simulink model "Control_Pc_prueba"  (R2021b)
settings: Solver=FixedStepDiscrete  StartTime=0.0  StopTime=inf  FixedStep=0.01  MaxStep=0.01  RelTol=1e-3
InitFcn:
  | Ts=0.01;
libraries: instrumentseriallib x2
settings Model: Creator=eva_g  LastModifiedBy=Laura Sierra Ruiz
settings SolverCC: AlgebraicLoopSolver=TrustRegion
settings DebuggingCC: SFMachineParentedDataDiag=warning

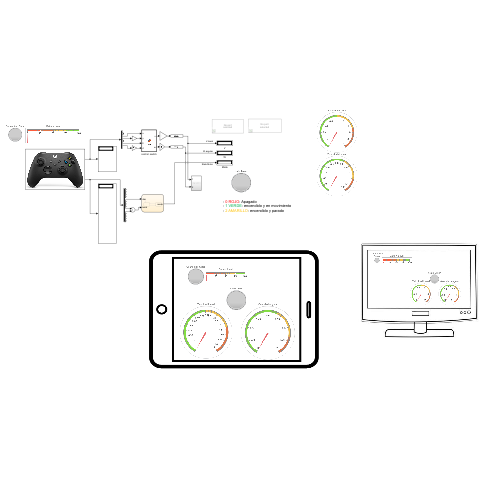
[thumbnail: Simulink's stored preview of the top-level diagram]
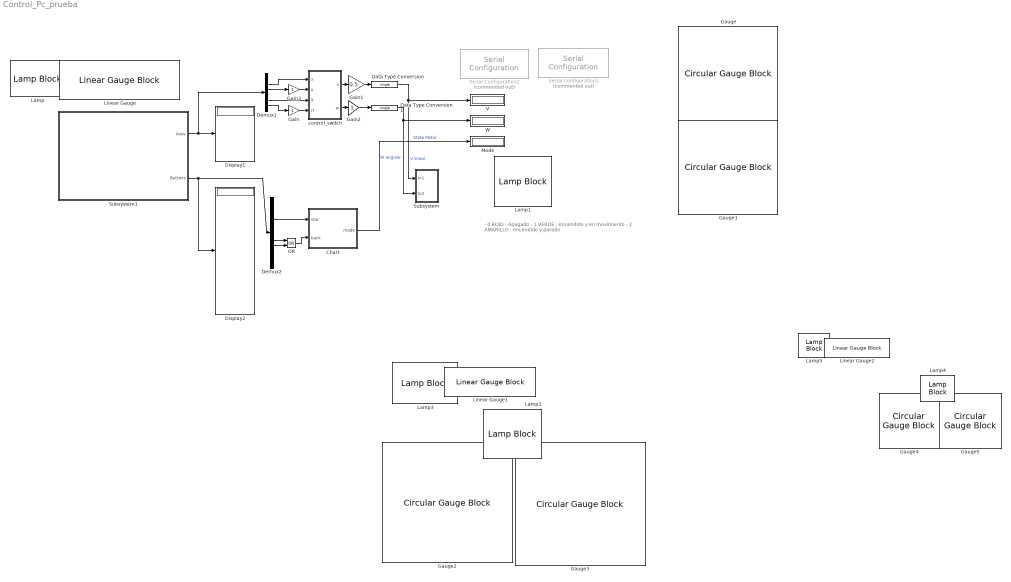
== system Control_Pc_prueba ==
  note: - 0 ROJO : Apagado
      | - 1 VERDE : encendido y en movimiento
      | - 2 AMARILLO : encendido y parado
  Chart : Stateflow chart  TreatAsAtomicUnit=on
  Data Type Conversion : DataTypeConversion  OutDataTypeStr=single
  Data Type Conversion1 : DataTypeConversion  OutDataTypeStr=single
  Demux1 : Demux  Outputs=6
  Demux2 : Demux  Outputs=14
  Display1 : Display
  Display2 : Display
  Gain : Gain  Gain=-1
  Gain1 : Gain  Gain=0.5
  Gain2 : Gain
  Gain3 : Gain  Gain=-1
  Gauge : CircularGaugeBlock  ScaleMax=2
  Gauge1 : CircularGaugeBlock  ScaleMax=1.2
  Gauge2 : CircularGaugeBlock  ScaleMax=2
  Gauge3 : CircularGaugeBlock  ScaleMax=1.2
  Gauge4 : CircularGaugeBlock  ScaleMax=2
  Gauge5 : CircularGaugeBlock  ScaleMax=1.2
  Lamp{,1..5} (6 alike) : LampBlock
  Linear Gauge : LinearGaugeBlock  TickInterval=25
  Linear Gauge1 : LinearGaugeBlock  TickInterval=25
  Linear Gauge2 : LinearGaugeBlock  TickInterval=25
  Mode : Display
  OR : Logic  Operator=OR  IconShape=distinctive  AllPortsSameDT=off  OutDataTypeStr=boolean
  Serial Configuration1 : instrumentseriallib/Serial Configuration  Priority=-200000  Commented=on  Port=<Select a port...>  ComPort=<Select a port...>  BaudRate=115200  DataBits=8  Parity=none  StopBits=1  ByteOrder=little-endian  FlowControl=none  Timeout=10  SimulateUsing=Interpreted execution  BlockInModel=on
  Serial Configuration2 : instrumentseriallib/Serial Configuration  Priority=-200000  Commented=on  Port=<Select a port...>  ComPort=<Select a port...>  BaudRate=115200  DataBits=8  Parity=none  StopBits=1  ByteOrder=little-endian  FlowControl=none  Timeout=10  SimulateUsing=Interpreted execution  BlockInModel=on
  Subsystem : Subsystem
  Subsystem1 : Subsystem
      mask Display: image('mando.PNG'); % Use "Edit Image" on toolstrip to change.
  V : Display
  W : Display
  control_switch : MATLAB Function  TreatAsAtomicUnit=on
  wires:
  Demux2/9 -> OR/1
  Gain1/1 -> Data Type Conversion/1
  Demux2/10 -> OR/2
  control_switch/1(v) -> Gain1/1
  Demux1/2 -> control_switch/1(x)
  Gain3/1 -> control_switch/2(y)
  control_switch/2(w) -> Gain2/1
  Demux2/5 -> Chart/1(star)
  Gain/1 -> control_switch/4(rt)
  Chart/1(mode) -> Mode/1  "State Motor"
  Demux1/3 -> Gain3/1
  Data Type Conversion1/1 -> W/1, Subsystem/2(In2)  "W angular"
  Gain2/1 -> Data Type Conversion1/1
  OR/1 -> Chart/2(back)
  Demux1/6 -> Gain/1
  Demux1/5 -> control_switch/3(lt)
  Data Type Conversion/1 -> Subsystem/1(In1), V/1  "V lineal"
  Subsystem1/2(Buttons) -> Display2/1, Demux2/1
  Subsystem1/1(Axes) -> Display1/1, Demux1/1

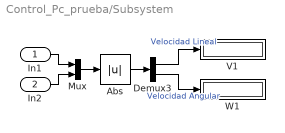
== system Control_Pc_prueba/Subsystem ==
  In1 : Inport
  In2 : Inport  Port=2
  Abs : Abs
  Demux3 : Demux  Outputs=2
  Mux : Mux  Inputs=2
  V1 : Display
  W1 : Display
  wires:
  Demux3/1 -> V1/1  "Velocidad Lineal"
  Mux/1 -> Abs/1
  Abs/1 -> Demux3/1
  In1/1 -> Mux/1
  Demux3/2 -> W1/1  "Velocidad Angular"
  In2/1 -> Mux/2

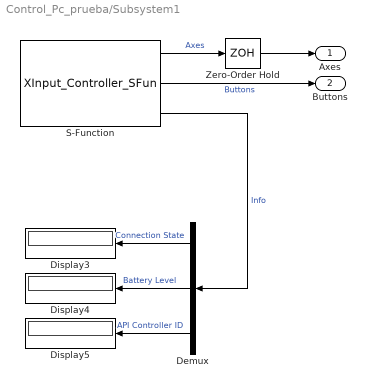
== system Control_Pc_prueba/Subsystem1 ==
  Demux : Demux  Outputs=3
  Display3 : Display
  Display4 : Display
  Display5 : Display
  S-Function : S-Function  FunctionName=XInput_Controller_SFun  Parameters=ControllerID  SFunctionDeploymentMode=off  EnableBusSupport=off  mask(XInput Controller){ControllerID=1}
      mask help:
      | This Block will allow you to use XInput Controllers in Simulink.
      | XInput is the most Supported API.
      | Works with XBOX 360 and XBOX ONE Controllers.
      |
      | Use 'DEMUX' to access Signals
      | Output_1 [1x6]
      |   Analog Left X, Analog Left Y,
      |   Analog Right X, Analog Right Y,
      |   Left Trigger, Right Trigger
      | Output_2 [1x14]
      |   Up, Down, Left, Right,
      |   Start, Back, Left Stick, Right Stick,
      |   Left Shoulder, Right Shoulder,
      |   A, B, X, Y
      | Output_3 [1x3]
      |   Connection State, Battery Level (1-4), Controller ID
      mask init:
      | ControllerID;   
      | blk = gcb; 
      | get_String = get_param(blk,'ControllerID');
      | ControllerID = str2double(get_String);
      mask Help:
      | Based on Microsoft XInput API
      | Therefore the maximum of conneced Gamepads per PC is 4. First Gamepad has Controller ID 1.
      | 
      | Reference:
      | https://docs.microsoft.com/en-us/windows/win32/api/_xinput/
      | 
      | Tutorial:
      | https://docs.microsoft.com/en-us/windows/win32/xinput/getting-started-with-xinput
      | 
      | Info:
      | The Analog Sticks Deadzone is coded to:
      | Deadzone = 6144;
      | 0 <= Deadzone <= 65534
      | This is smaller then Microsoft default.
      | 
      | created by Mathias Voigt
      | Technische Universität Dresden
      | 2019
      mask TypeOptions ControllerID: 1 | 2 | 3 | 4
      mask DialogControl ParameterGroupVar Prompt: Controller ID
      mask Display:
      | %% Set Block picture from user Data
      | %  (permanent, picture file not needed)
      | %  see persistent_image_allocation.m
      | 
      | %get the picture data
      | UserDataStrut = get_param(gcb, 'UserData');
      | image(UserDataStrut.Image, [0.2, 0.3, 0.6, 0.6])
      | 
      | 
      | 
      | % conventional method (does not save picture data in Simulink)
      | % image('XBOX_One_Controller_Icon.png', [0.2, 0.3, 0.6, 0.6])
      | 
      | %% Create Port Labels
      | color('blue');
      | port_label('output', 1, 'Axes');
      | port_label('output', 2, 'Buttons');
      | port_label('output', 3, 'Info');
      | 
      | 
      | %% Create S-Function Block Name
      | color('black');
      | text(0.5, 0.1, 'XInput Controller',...
      |      'horizontalAlignment', 'center',...
      |      'verticalAlignment', 'bottom');
  Zero-Order Hold : ZeroOrderHold  SampleTime=-1
  Axes : Outport
  Buttons : Outport  Port=2
  wires:
  Demux/1 -> Display3/1  "Connection State"
  Demux/2 -> Display4/1  "Battery Level"
  Zero-Order Hold/1 -> Axes/1
  Demux/3 -> Display5/1  "API Controller ID"
  S-Function/1 -> Zero-Order Hold/1  "Axes"
  S-Function/3 -> Demux/1  "Info"
  S-Function/2 -> Buttons/1  "Buttons"

== stateflow chart Control_Pc_prueba/Chart ==
  state ON
    entry: mode=1;
  state OFF
    entry: mode=0;
  (default) -> OFF
  ON -> OFF : [back>0]
  OFF -> ON : [star>0]
  data: mode output; star input; back input

== matlab function Control_Pc_prueba/control_switch ==
  data: x input; v output; y input; lt input; rt input; w output
function [v,w]=fcn(x,y,lt,rt)

    if (rt==0) && (lt==0) && ((x>=0.3) || (x<=-0.3))
        v=x;
        w=y;
    elseif (x~=0) && ((rt~=0) || (lt~=0))
        w=0;
        v=0;
    elseif (x==0) && (y==0) && (rt==0) && (lt~=0)
        w=lt;
        v=0;
    elseif (x==0) && (y==0) && (lt==0) && (rt~=0)
        w=rt;
        v=0;
    elseif (lt~=0) && (rt~=0)
        w=0;
        v=0;
    elseif (x==0) || (y==0) || (lt==0) 
        w=lt;
        v=0;
    else
        w=0;
        v=0;
    end;
